simulink model "SCARA"  (R2020b)
settings: Solver=VariableStepAuto  StartTime=0.0  StopTime=20  RelTol=1e-3
settings Model: Creator=hp  LastModifiedBy=hp
settings DataIOCC: ReturnWorkspaceOutputs=off
settings DebuggingCC: ArithmeticOperatorsInVariantConditions=warning
settings SFSimCC: SimUseLocalCustomCode=off  CustomCodeUndefinedFunction=UseInterfaceOnly
settings RTWCC: RTWUseLocalCustomCode=off

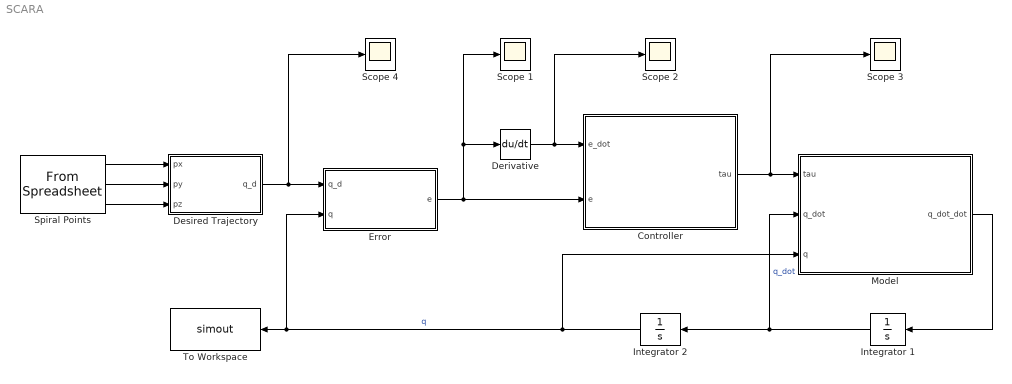
== system SCARA ==
  Controller : MATLAB Function  TreatAsAtomicUnit=on
  Derivative : Derivative
  Desired Trajectory : MATLAB Function  TreatAsAtomicUnit=on
  Error : MATLAB Function  TreatAsAtomicUnit=on
  Integrator 1 : Integrator  InitialCondition=[0;0;0;0]
  Integrator 2 : Integrator  InitialCondition=[0;0;0;0]
  Model : MATLAB Function  TreatAsAtomicUnit=on
  Scope {1..4} (4 alike) : Scope
  Spiral Points : FromSpreadsheet  FileName=Waypoints.xlsx  OutDataTypeStr=double
  To Workspace : ToWorkspace  VariableName=simout  SampleTime=-1
  wires:
  Desired Trajectory/1(q_d) -> Scope 4/1, Error/1(q_d)
  Error/1(e) -> Controller/2(e), Scope 1/1, Derivative/1
  Derivative/1 -> Scope 2/1, Controller/1(e_dot)
  Controller/1(tau) -> Scope 3/1, Model/1(tau)
  Model/1(q_dot_dot) -> Integrator 1/1
  Integrator 1/1 -> Model/2(q_dot), Integrator 2/1  "q_dot"
  Integrator 2/1 -> Model/3(q), Error/2(q), To Workspace/1  "q"
  Spiral Points/1 -> Desired Trajectory/1(px)
  Spiral Points/2 -> Desired Trajectory/2(py)
  Spiral Points/3 -> Desired Trajectory/3(pz)

== matlab function SCARA/Error ==
  data: q_d input; q input; e output
function e = fcn(q_d,q)

e = q - q_d;

end

== matlab function SCARA/Desired Trajectory ==
  data: px input; py input; pz input; q_d output
function q_d = fnc(px,py,pz)

a1=0.2; a2=0.25;

theta2 = acos( ( (px*px)+(py*py)-(a1*a1)-(a2*a2) )/(2*a1*a2) );  %% Multiple solutions because cos(-theta) = cos(theta)

k1 = a1+(a2*cos(theta2));
k2 = a2*sin(theta2);

theta1 = atan( ((k1*py)-(k2*px))/((k1*px)+(k2*py)) );
theta3 = 0;
d4 = -pz;

q_d = [ theta1;  
        theta2;
        theta3;
          d4 ];   
      
end

== matlab function SCARA/Controller ==
  data: e_dot input; e input; tau output
function tau = fcn(e_dot,e)

k1=2500;
k2=175;
tau = -(k1*e)-(k2*e_dot);

end

== matlab function SCARA/Model ==
  data: tau input; q_dot_dot output; q_dot input; q input
function q_dot_dot  = fcn(tau,q_dot,q)

m1=20; m2=15; m3=15; m4=0.5; l1=0.2; l2=0.25; g=9.8;
r1=0.1; r2=0.125; Iz1=0.27; Iz2=0.31; Iz3=0.02; Iz4=0.0001;
    
theta1_dot=q_dot(1,1); theta2_dot=q_dot(2,1);
theta2=q(2,1);

alpha = Iz1+(r1*r1*m1)+(l1*l1*m2)+(l1*l1*m3)+(l1*l1*m4);
beta = Iz1+Iz2+Iz3+Iz4+(l2*l2*m3)+(l2*l2*m4)+(r2*r2*m2);
gamma = (l1*l2*m3)+(l1*l2*m4)+(l1*m2*r2);
psi = Iz3+Iz4;

mass_matrix = [ alpha+beta+(2*gamma*cos(theta2)), beta+(gamma*cos(theta2)), psi, 0 ;
                beta+(gamma*cos(theta2))        , beta                    , psi, 0 ;
                psi                             , psi                     , psi, 0 ;
                0                               , 0                       , 0  , m4 ];
             
coriolis_term = [ -gamma*sin(theta2)*theta2_dot, -gamma*sin(theta2)*(theta1_dot+theta2_dot),0 ,0 ;
                  -gamma*sin(theta2)*theta1_dot, 0                                         ,0 ,0 ;
                   0                           , 0                                         ,0 ,0 ;
                   0                           , 0                                         ,0 ,0 ];
                              
gravity_term = [ 0 ;
                 0 ;
                 0 ;
                 m4*g ];
              
q_dot_dot = mass_matrix \ (tau-coriolis_term*q_dot-gravity_term);           
                                                                                        
end
